simulink model "NGIL_Controller"  (R2024a)
settings: Solver=FixedStepDiscrete  StartTime=0.0  StopTime=1  FixedStep=0.001  RelTol=1e-3
InitFcn:
  | addpath(fileparts(fileparts(get_param(bdroot,'FileName')))); setup;
undefined symbols (not defined in the file): base_slip
libraries: simulink_extras x5
settings Model: Creator=fangr  LastModifiedBy=fangr
settings DataIOCC: SignalLogging=off

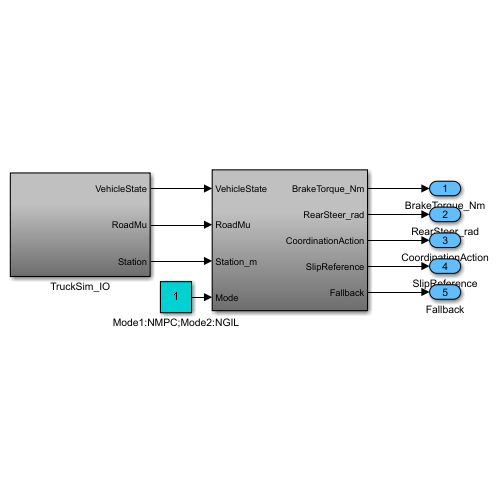
[thumbnail: Simulink's stored preview of the top-level diagram]
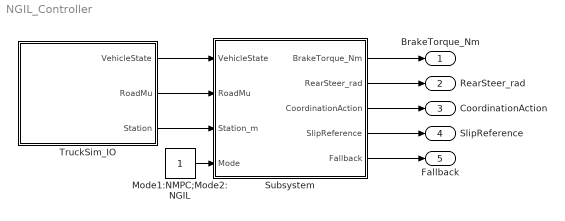
== system NGIL_Controller ==
  Mode1:NMPC;Mode2:NGIL : Constant
  Subsystem : Subsystem
  TruckSim_IO : Subsystem
  BrakeTorque_Nm : Outport
  RearSteer_rad : Outport  Port=2
  CoordinationAction : Outport  Port=3
  SlipReference : Outport  Port=4
  Fallback : Outport  Port=5
  wires:
  Subsystem/5(Fallback) -> Fallback/1
  Subsystem/4(SlipReference) -> SlipReference/1
  Subsystem/3(CoordinationAction) -> CoordinationAction/1
  Subsystem/2(RearSteer_rad) -> RearSteer_rad/1
  Subsystem/1(BrakeTorque_Nm) -> BrakeTorque_Nm/1
  TruckSim_IO/1(VehicleState) -> Subsystem/1(VehicleState)
  TruckSim_IO/2(RoadMu) -> Subsystem/2(RoadMu)
  TruckSim_IO/3(Station) -> Subsystem/3(Station_m)
  Mode1:NMPC;Mode2:NGIL/1 -> Subsystem/4(Mode)

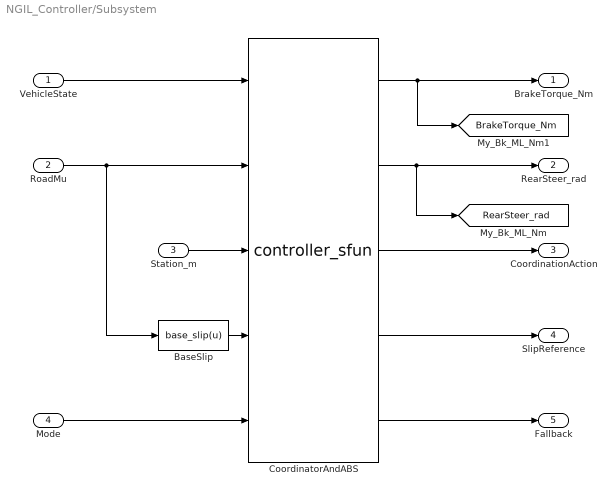
== system NGIL_Controller/Subsystem ==
  VehicleState : Inport  OutDataTypeStr=double  PortDimensions=12  SampleTime=0.001  Interpolate=off
  RoadMu : Inport  Port=2  OutDataTypeStr=double  PortDimensions=2  SampleTime=0.001  Interpolate=off
  Station_m : Inport  Port=3  OutDataTypeStr=double  PortDimensions=1  SampleTime=0.001  Interpolate=off
  Mode : Inport  Port=4  OutDataTypeStr=double  PortDimensions=1  SampleTime=0.001  Interpolate=off
  BaseSlip : MATLABFcn  MATLABFcn=base_slip(u)  OutputDimensions=6
  CoordinatorAndABS : M-S-Function  FunctionName=controller_sfun
  BrakeTorque_Nm : Outport
  RearSteer_rad : Outport  Port=2
  CoordinationAction : Outport  Port=3
  SlipReference : Outport  Port=4
  Fallback : Outport  Port=5
  tag scope: BrakeTorque_Nm=global, RearSteer_rad=global
  wires:
  BaseSlip/1 -> CoordinatorAndABS/4
  CoordinatorAndABS/2 -> [RearSteer_rad], RearSteer_rad/1
  CoordinatorAndABS/5 -> Fallback/1
  CoordinatorAndABS/1 -> [BrakeTorque_Nm], BrakeTorque_Nm/1
  CoordinatorAndABS/4 -> SlipReference/1
  CoordinatorAndABS/3 -> CoordinationAction/1
  Mode/1 -> CoordinatorAndABS/5
  Station_m/1 -> CoordinatorAndABS/3
  RoadMu/1 -> BaseSlip/1, CoordinatorAndABS/2
  VehicleState/1 -> CoordinatorAndABS/1

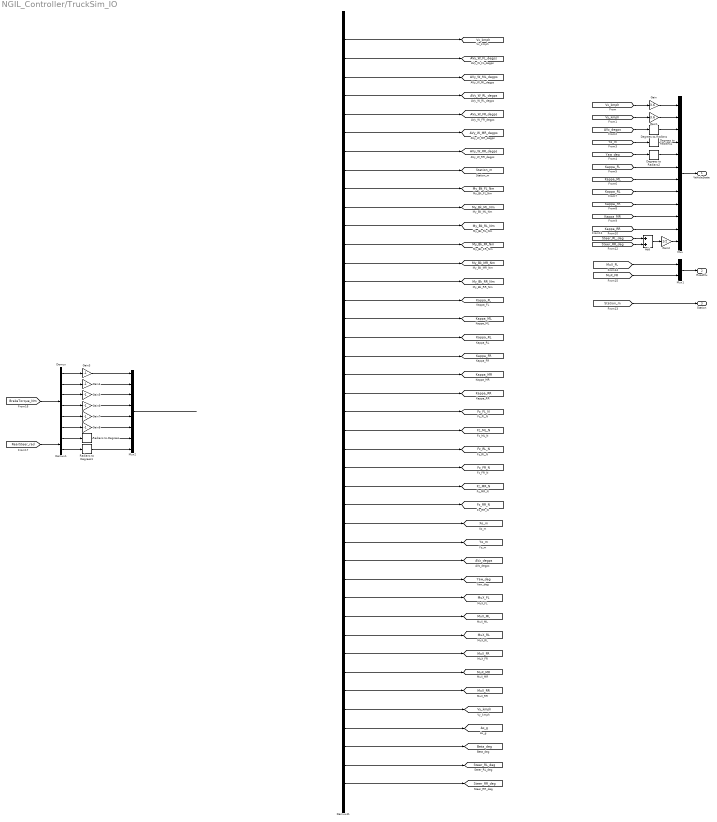
== system NGIL_Controller/TruckSim_IO ==
  Add : Sum
  Degrees to Radians : simulink_extras/Transformations/Degrees to Radians
  Degrees to Radians1 : simulink_extras/Transformations/Degrees to Radians
  Degrees to Radians2 : simulink_extras/Transformations/Degrees to Radians
  Demux : Demux  Outputs=6
  Demux1 : Demux  Outputs=2
  Demux41 : Demux  Outputs=41
  Gain : Gain  Gain=3.6
  Gain1 : Gain  Gain=3.6
  Gain2 : Gain  Gain=1/2
  Gain{3..8} (6 alike) : Gain  Gain=-1
  Mux : Mux  Inputs=12
  Mux1 : Mux  Inputs=2
  Mux2 : Mux  Inputs=8
  Radians to Degrees : simulink_extras/Transformations/Radians to Degrees
  Radians to Degrees1 : simulink_extras/Transformations/Radians to Degrees
  VehicleState : Outport
  RoadMu : Outport  Port=2
  Station : Outport  Port=3
  tag scope: AVy_W_FL_degps=global, AVy_W_FR_degps=global, AVy_W_ML_degps=global, AVy_W_MR_degps=global, AVy_W_RL_degps=global, AVy_W_RR_degps=global, AVz_degps=global, Ax_g=global, Beta_deg=global, Fz_FL_N=global, Fz_FR_N=global, Fz_ML_N=global, Fz_MR_N=global, Fz_RL_N=global, Fz_RR_N=global, Kappa_FL=global, Kappa_FR=global, Kappa_ML=global, Kappa_MR=global, Kappa_RL=global, Kappa_RR=global, MuX_FL=global, MuX_FR=global, MuX_ML=global, MuX_MR=global, MuX_RL=global, MuX_RR=global, My_Bk_FL_Nm=global, My_Bk_FR_Nm=global, My_Bk_ML_Nm=global, My_Bk_MR_Nm=global, My_Bk_RL_Nm=global, My_Bk_RR_Nm=global, Station_m=global, Steer_RL_deg=global, Steer_RR_deg=global, Vx_kmph=global, Vy_kmph=global, Xo_m=global, Yaw_deg=global, Yo_m=global
  wires:
  Demux41/3 -> [AVy_W_ML_degps]
  Demux41/6 -> [AVy_W_MR_degps]
  Demux41/1 -> [Vx_kmph]
  Demux41/5 -> [AVy_W_FR_degps]
  Demux41/4 -> [AVy_W_RL_degps]
  Demux41/35 -> [MuX_MR]
  Demux41/34 -> [MuX_FR]
  Demux41/2 -> [AVy_W_FL_degps]
  Demux41/11 -> [My_Bk_RL_Nm]
  Demux41/10 -> [My_Bk_ML_Nm]
  Demux41/7 -> [AVy_W_RR_degps]
  Demux41/8 -> [Station_m]
  Demux41/9 -> [My_Bk_FL_Nm]
  Demux41/12 -> [My_Bk_FR_Nm]
  Demux41/13 -> [My_Bk_MR_Nm]
  Demux41/15 -> [Kappa_FL]
  Demux41/14 -> [My_Bk_RR_Nm]
  Demux41/17 -> [Kappa_RL]
  Demux41/16 -> [Kappa_ML]
  Demux41/37 -> [Vy_kmph]
  Demux41/36 -> [MuX_RR]
  Demux41/19 -> [Kappa_MR]
  Demux41/18 -> [Kappa_FR]
  Demux41/39 -> [Beta_deg]
  Demux41/38 -> [Ax_g]
  Demux41/21 -> [Fz_FL_N]
  Demux41/20 -> [Kappa_RR]
  Demux41/22 -> [Fz_ML_N]
  Demux41/23 -> [Fz_RL_N]
  Demux41/25 -> [Fz_MR_N]
  Demux41/24 -> [Fz_FR_N]
  Demux41/27 -> [Xo_m]
  Demux41/26 -> [Fz_RR_N]
  Demux41/29 -> [AVz_degps]
  Demux41/28 -> [Yo_m]
  Demux41/31 -> [MuX_FL]
  Demux41/30 -> [Yaw_deg]
  Demux41/33 -> [MuX_RL]
  Demux41/32 -> [MuX_ML]
  Demux41/41 -> [Steer_RR_deg]
  Demux41/40 -> [Steer_RL_deg]
  ? -> Demux41/1
  [Steer_RR_deg] -> Add/2
  Gain/1 -> Mux/1
  Gain1/1 -> Mux/2
  Degrees to Radians/1 -> Mux/3
  [Kappa_FL] -> Mux/6
  Degrees to Radians2/1 -> Mux/5
  Degrees to Radians1/1 -> Mux/4
  Add/1 -> Gain2/1
  [Kappa_RL] -> Mux/8
  [Kappa_ML] -> Mux/7
  [Kappa_MR] -> Mux/10
  [Kappa_FR] -> Mux/9
  [Vx_kmph] -> Gain/1
  Gain2/1 -> Mux/12
  [Kappa_RR] -> Mux/11
  [AVz_degps] -> Degrees to Radians/1
  Mux/1 -> VehicleState/1
  [Yo_m] -> Degrees to Radians1/1
  [Vy_kmph] -> Gain1/1
  [Yaw_deg] -> Degrees to Radians2/1
  [Steer_RL_deg] -> Add/1
  Mux1/1 -> RoadMu/1
  [MuX_FL] -> Mux1/1
  [MuX_FR] -> Mux1/2
  [Station_m] -> Station/1
  [BrakeTorque_Nm] -> Demux/1
  Demux/5 -> Gain7/1
  Demux/6 -> Gain8/1
  Demux/4 -> Gain6/1
  Demux/3 -> Gain5/1
  Demux/2 -> Gain4/1
  Demux/1 -> Gain3/1
  [RearSteer_rad] -> Demux1/1
  Demux1/1 -> Radians to Degrees/1
  Demux1/2 -> Radians to Degrees1/1
  Gain4/1 -> Mux2/2
  Gain5/1 -> Mux2/3
  Gain3/1 -> Mux2/1
  Gain6/1 -> Mux2/4
  Gain7/1 -> Mux2/5
  Gain8/1 -> Mux2/6
  Radians to Degrees/1 -> Mux2/7
  Radians to Degrees1/1 -> Mux2/8
  Mux2/1 -> ?
